simulink model "invPendulum"  (R2025b)
settings: Solver=FixedStepAuto  StartTime=0.0  StopTime=20  FixedStep=0.01  RelTol=1e-3
model workspace (MAT data in the model file):
  M = 2.4
  dtheta0 = 0
  dx0 = 0
  g = 9.8
  l = 0.36
  m = 0.23
  theta0 = 10
  x0 = 0
libraries: simulink_extras x2
settings Model: Creator=votua  LastModifiedBy=votua

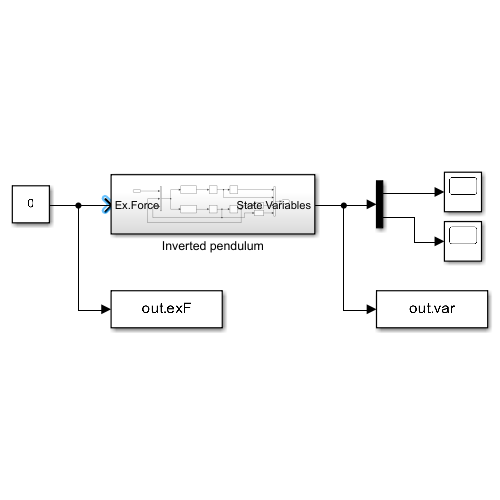
[thumbnail: Simulink's stored preview of the top-level diagram]
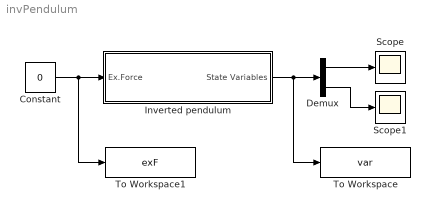
== system invPendulum ==
  Constant : Constant  Value=0
  Demux : Demux  Outputs=2
  Inverted pendulum : Subsystem
  Scope : Scope
      settings: ActiveDisplayYMinimum=-0.56593974246722034  ActiveDisplayYMaximum=0.41393535331880615
  Scope1 : Scope
      settings: ActiveDisplayYMinimum=-253.8042053051297  ActiveDisplayYMaximum=635.18337703157624
  To Workspace : ToWorkspace  VariableName=var  SaveFormat=Timeseries  SampleTime=-1
  To Workspace1 : ToWorkspace  VariableName=exF  SaveFormat=Timeseries  SampleTime=-1
  wires:
  Inverted pendulum/1(State Variables) -> To Workspace/1, Demux/1
  Constant/1 -> To Workspace1/1, Inverted pendulum/1(Ex.Force)
  Demux/1 -> Scope/1
  Demux/2 -> Scope1/1

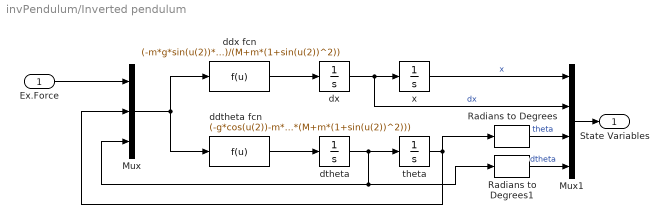
== system invPendulum/Inverted pendulum ==
  Ex.Force : Inport
  Mux : Mux  Inputs=3
  Mux1 : Mux
  Radians to Degrees : simulink_extras/Transformations/Radians to Degrees
  Radians to Degrees1 : simulink_extras/Transformations/Radians to Degrees
  ddtheta fcn : Fcn  Expr=(-g*cos(u(2))-m*l*cos(u(2))*sin(u(2))*u(3)^2+u(1)*sin(u(2)))/(l*(M+m*(1+sin(u(2))^2)))
  ddx fcn : Fcn  Expr=(-m*g*sin(u(2))*cos(u(2))-m*l*cos(u(2))*u(3)^2+u(1))/(M+m*(1+sin(u(2))^2))
  dtheta : Integrator  InitialCondition=deg2rad(dtheta0)
  dx : Integrator  InitialCondition=dx0
  theta : Integrator  InitialCondition=deg2rad(theta0) + pi/2
  x : Integrator  InitialCondition=x0
  State Variables : Outport
  wires:
  ddtheta fcn/1 -> dtheta/1
  dtheta/1 -> Radians to Degrees1/1, Mux/3, theta/1
  ddx fcn/1 -> dx/1
  Ex.Force/1 -> Mux/1
  Mux/1 -> ddx fcn/1, ddtheta fcn/1
  dx/1 -> Mux1/2, x/1  "dx"
  Mux1/1 -> State Variables/1
  x/1 -> Mux1/1  "x"
  theta/1 -> Mux/2, Radians to Degrees/1
  Radians to Degrees/1 -> Mux1/3  "theta"
  Radians to Degrees1/1 -> Mux1/4  "dtheta"
